simulink model "stable_ctime_v5"  (R2012b)
settings: Solver=VariableStepDiscrete  SolverMode=SingleTasking  StartTime=0.0  StopTime=10.0  RelTol=1e-3
undefined symbols (not defined in the file): pfb_coeff_gen_calc
libraries: xbsIndex_r4 x5705, casper_library_misc x63, casper_library_delays x27, casper_library_flow_control x20, xps_library x6
(part 2 of 68)

== system stable_ctime_v5/DAC_ADC ==
  i0 : Inport
  i1 : Inport  Port=2
  q0 : Inport  Port=3
  q1 : Inport  Port=4
  sync_iq : Inport  Port=5
  dac_reset : Inport  Port=6
  adc_mkid : xps_library/ADCs/adc_mkid  Tag=xps:adc_mkid  adc_brd=1  adc_clk_rate=512
  dac_mkid1 : Subsystem  Tag=xps:dac_mkid  AncestorBlock=xps_library/DACs/dac_mkid  mask(MKID DAC Interface Block){dac_brd=0, dac_clk_rate=512, sample_period=1}
      mask prompts: dac_brd "DAC board"; dac_clk_rate "DAC external clock rate (MHz)"; sample_period "Sample period"
      mask help: Interface block for the MKID 16-bits DAC board (2xDAC5681)
      mask init:
      | dac_mkid_mask;
      mask TypeOptions dac_brd: 0 | 1
  i0_adc : Outport
  i1_adc : Outport  Port=2
  q0_adc : Outport  Port=3
  q1_adc : Outport  Port=4
  sync : Outport  Port=5
  wires:
  i0/1 -> dac_mkid1/1(data_i0)
  i1/1 -> dac_mkid1/2(data_i1)
  q1/1 -> dac_mkid1/4(data_q1)
  adc_mkid/5 -> sync/1
  adc_mkid/2 -> i1_adc/1
  adc_mkid/4 -> q1_adc/1
  q0/1 -> dac_mkid1/3(data_q0)
  adc_mkid/3 -> q0_adc/1
  adc_mkid/1 -> i0_adc/1
  dac_reset/1 -> dac_mkid1/7(reset)
  sync_iq/1 -> dac_mkid1/6(sync_q), dac_mkid1/5(sync_i)

== system stable_ctime_v5/DDC ==
  note: latency = 8
  "sync_in " : Inport
  i0q0 : Inport  Port=2
  i1q1 : Inport  Port=3
  dds_delay : Inport  Port=4
  dds_i0 : Inport  Port=5
  "dds_q0 " : Inport  Port=6
  dds_i1 : Inport  Port=7
  dds_q1 : Inport  Port=8
  Delay{1,34..37} (5 alike) : xbsIndex_r4/Delay  rst=off  infoeditControl=Selection of Reset will increase slice count due to use of real FFs and instead of SRLs  en=off  latency=2  dbl_ovrd=off  reg_retiming=off  block_type=delay
  Delay2 : xbsIndex_r4/Delay  rst=off  infoeditControl=Selection of Reset will increase slice count due to use of real FFs and instead of SRLs  en=off  latency=8  dbl_ovrd=off  reg_retiming=off  block_type=delay
  c_to_ri3 : casper_library_misc/c_to_ri  n_bits=18  bin_pt=17
  c_to_ri6 : casper_library_misc/c_to_ri  n_bits=18  bin_pt=17
  delay_bram_prog : casper_library_delays/delay_bram_prog  MaxDelay=9  bram_latency=2
      link override AddSub: mode=Subtraction  use_carryin=off  use_carryout=off  en=off  latency=2  precision=User Defined  arith_type=Unsigned  n_bits=MaxDelay  bin_pt=0  quantization=Truncate  overflow=Wrap  dbl_ovrd=off  use_behavioral_HDL=off  hw_selection=DSP48  pipelined=on  use_rpm=on
      link override Counter: cnt_type=Free Running  cnt_to=inf  operation=Up  start_count=0  cnt_by_val=1  arith_type=Unsigned  n_bits=MaxDelay  bin_pt=0  load_pin=off  rst=on  en=off  explicit_period=on  period=1  dbl_ovrd=off  use_behavioral_HDL=off  implementation=DSP48  use_rpm=off
      link override Relational: mode=a>=b  en=off  latency=0  dbl_ovrd=off
      link override Single Port RAM: depth=2^MaxDelay  initVector=0  distributed_mem=Block RAM  write_mode=Read Before Write  rst=off  init_reg=0  en=off  latency=bram_latency  dbl_ovrd=off  optimize=Speed
      link override AddSub: xl_area=[0, 0, 0, 0, 0, 0, 0]
      link override Counter: infoedit="Hardware notes: Free running counters are the least expensive in hardware.  A count limited counter is implemented by combining a counter with a comparator."  xl_area=[0, 0, 0, 0, 0, 0, 0]
      link override Relational: xl_area=[0, 0, 0, 0, 0, 0, 0]
      link override Single Port RAM: xl_area=[0, 0, 0, 0, 0, 0, 0]
  delay_bram_prog1 : casper_library_delays/delay_bram_prog  MaxDelay=9  bram_latency=2
      link override AddSub: mode=Subtraction  use_carryin=off  use_carryout=off  en=off  latency=2  precision=User Defined  arith_type=Unsigned  n_bits=MaxDelay  bin_pt=0  quantization=Truncate  overflow=Wrap  dbl_ovrd=off  use_behavioral_HDL=off  hw_selection=DSP48  pipelined=on  use_rpm=on
      link override Counter: cnt_type=Free Running  cnt_to=inf  operation=Up  start_count=0  cnt_by_val=1  arith_type=Unsigned  n_bits=MaxDelay  bin_pt=0  load_pin=off  rst=on  en=off  explicit_period=on  period=1  dbl_ovrd=off  use_behavioral_HDL=off  implementation=DSP48  use_rpm=off
      link override Relational: mode=a>=b  en=off  latency=0  dbl_ovrd=off
      link override Single Port RAM: depth=2^MaxDelay  initVector=0  distributed_mem=Block RAM  write_mode=Read Before Write  rst=off  init_reg=0  en=off  latency=bram_latency  dbl_ovrd=off  optimize=Speed
      link override AddSub: xl_area=[0, 0, 0, 0, 0, 0, 0]
      link override Counter: infoedit="Hardware notes: Free running counters are the least expensive in hardware.  A count limited counter is implemented by combining a counter with a comparator."  xl_area=[0, 0, 0, 0, 0, 0, 0]
      link override Relational: xl_area=[0, 0, 0, 0, 0, 0, 0]
      link override Single Port RAM: xl_area=[0, 0, 0, 0, 0, 0, 0]
  delay_bram_prog2 : casper_library_delays/delay_bram_prog  MaxDelay=9  bram_latency=2
      link override AddSub: mode=Subtraction  use_carryin=off  use_carryout=off  en=off  latency=2  precision=User Defined  arith_type=Unsigned  n_bits=MaxDelay  bin_pt=0  quantization=Truncate  overflow=Wrap  dbl_ovrd=off  use_behavioral_HDL=off  hw_selection=DSP48  pipelined=on  use_rpm=on
      link override Counter: cnt_type=Free Running  cnt_to=inf  operation=Up  start_count=0  cnt_by_val=1  arith_type=Unsigned  n_bits=MaxDelay  bin_pt=0  load_pin=off  rst=on  en=off  explicit_period=on  period=1  dbl_ovrd=off  use_behavioral_HDL=off  implementation=DSP48  use_rpm=off
      link override Relational: mode=a>=b  en=off  latency=0  dbl_ovrd=off
      link override Single Port RAM: depth=2^MaxDelay  initVector=0  distributed_mem=Block RAM  write_mode=Read Before Write  rst=off  init_reg=0  en=off  latency=bram_latency  dbl_ovrd=off  optimize=Speed
      link override AddSub: xl_area=[0, 0, 0, 0, 0, 0, 0]
      link override Counter: infoedit="Hardware notes: Free running counters are the least expensive in hardware.  A count limited counter is implemented by combining a counter with a comparator."  xl_area=[0, 0, 0, 0, 0, 0, 0]
      link override Relational: xl_area=[0, 0, 0, 0, 0, 0, 0]
      link override Single Port RAM: xl_area=[0, 0, 0, 0, 0, 0, 0]
  delay_bram_prog3 : casper_library_delays/delay_bram_prog  MaxDelay=9  bram_latency=2
      link override AddSub: mode=Subtraction  use_carryin=off  use_carryout=off  en=off  latency=2  precision=User Defined  arith_type=Unsigned  n_bits=MaxDelay  bin_pt=0  quantization=Truncate  overflow=Wrap  dbl_ovrd=off  use_behavioral_HDL=off  hw_selection=DSP48  pipelined=on  use_rpm=on
      link override Counter: cnt_type=Free Running  cnt_to=inf  operation=Up  start_count=0  cnt_by_val=1  arith_type=Unsigned  n_bits=MaxDelay  bin_pt=0  load_pin=off  rst=on  en=off  explicit_period=on  period=1  dbl_ovrd=off  use_behavioral_HDL=off  implementation=DSP48  use_rpm=off
      link override Relational: mode=a>=b  en=off  latency=0  dbl_ovrd=off
      link override Single Port RAM: depth=2^MaxDelay  initVector=0  distributed_mem=Block RAM  write_mode=Read Before Write  rst=off  init_reg=0  en=off  latency=bram_latency  dbl_ovrd=off  optimize=Speed
      link override AddSub: xl_area=[0, 0, 0, 0, 0, 0, 0]
      link override Counter: infoedit="Hardware notes: Free running counters are the least expensive in hardware.  A count limited counter is implemented by combining a counter with a comparator."  xl_area=[0, 0, 0, 0, 0, 0, 0]
      link override Relational: xl_area=[0, 0, 0, 0, 0, 0, 0]
      link override Single Port RAM: xl_area=[0, 0, 0, 0, 0, 0, 0]
  mixer_even : Subsystem
  mixer_odd : Subsystem
  "sync_out " : Outport
  i0q0_out : Outport  Port=2
  i1q1_out : Outport  Port=3
  wires:
  i1q1/1 -> c_to_ri6/1
  i0q0/1 -> c_to_ri3/1
  dds_delay/1 -> delay_bram_prog1/2, delay_bram_prog3/2, delay_bram_prog2/2, delay_bram_prog/2
  c_to_ri3/1 -> Delay36/1
  c_to_ri3/2 -> Delay37/1
  c_to_ri6/1 -> Delay34/1
  c_to_ri6/2 -> Delay35/1
  dds_i0/1 -> delay_bram_prog/1
  delay_bram_prog/1 -> mixer_even/3(dds_I)
  "dds_q0 "/1 -> delay_bram_prog1/1
  dds_q1/1 -> delay_bram_prog3/1
  delay_bram_prog3/1 -> mixer_odd/4(dds_Q)
  delay_bram_prog1/1 -> mixer_even/4(dds_Q)
  Delay35/1 -> mixer_odd/2(data_Q)
  Delay34/1 -> mixer_odd/1(data_I)
  Delay36/1 -> mixer_even/1(data_I)
  Delay37/1 -> mixer_even/2(data_Q)
  delay_bram_prog2/1 -> mixer_odd/3(dds_I)
  mixer_even/1(mixed_out) -> i0q0_out/1
  mixer_odd/1(mixed_out) -> i1q1_out/1
  dds_i1/1 -> delay_bram_prog2/1
  "sync_in "/1 -> Delay1/1
  Delay1/1 -> Delay2/1
  Delay2/1 -> "sync_out "/1

== system stable_ctime_v5/DDC_snap ==
  note: 18.17 to 16.15
  sync_in : Inport
  i0q0_fft : Inport  Port=2
  i1q1_fft : Inport  Port=3
  i0q0_ddc : Inport  Port=4
  i1q1_ddc : Inport  Port=5
  dds_shift : Inport  Port=6
  dds_i0 : Inport  Port=7
  dds_q0 : Inport  Port=8
  dds_i1 : Inport  Port=9
  dds_q1 : Inport  Port=10
  Counter2 : xbsIndex_r4/Counter  cnt_type=Free Running  cnt_to=Inf  operation=Up  start_count=0  cnt_by_val=1  arith_type=Unsigned  n_bits=9  bin_pt=0  load_pin=off  rst=on  en=off  explicit_period=on  period=1  dbl_ovrd=off  use_behavioral_HDL=off  implementation=DSP48  block_type=counter
  Delay17 : xbsIndex_r4/Delay  rst=off  infoeditControl=Selection of Reset will increase slice count due to use of real FFs and instead of SRLs  en=off  latency=2  dbl_ovrd=off  reg_retiming=off  block_type=delay
  Delay25 : xbsIndex_r4/Delay  rst=off  infoeditControl=Selection of Reset will increase slice count due to use of real FFs and instead of SRLs  en=off  latency=2  dbl_ovrd=off  reg_retiming=off  block_type=delay
  Delay39 : xbsIndex_r4/Delay  rst=off  infoeditControl=Selection of Reset will increase slice count due to use of real FFs and instead of SRLs  en=off  latency=2  dbl_ovrd=off  reg_retiming=off  block_type=delay
  Delay42 : xbsIndex_r4/Delay  rst=off  infoeditControl=Selection of Reset will increase slice count due to use of real FFs and instead of SRLs  en=off  latency=8  dbl_ovrd=off  reg_retiming=off  block_type=delay
  Relational1 : xbsIndex_r4/Relational  mode=a=b  en=off  latency=0  dbl_ovrd=off  block_type=relational
  bus_create6 : Subsystem  AncestorBlock=casper_library_flow_control/bus_create  mask(bus_create){inputNum=4}
      mask prompts: inputNum "Number of inputs:"
      mask init:
      | bus_create_init(gcb,...
      |     'inputNum', inputNum);
  bus_create7 : Subsystem  AncestorBlock=casper_library_flow_control/bus_create  mask(bus_create){inputNum=2}
      mask prompts: inputNum "Number of inputs:"
      mask init:
      | bus_create_init(gcb,...
      |     'inputNum', inputNum);
  bus_create8 : Subsystem  AncestorBlock=casper_library_flow_control/bus_create  mask(bus_create){inputNum=2}
      mask prompts: inputNum "Number of inputs:"
      mask init:
      | bus_create_init(gcb,...
      |     'inputNum', inputNum);
  bus_create9 : Subsystem  AncestorBlock=casper_library_flow_control/bus_create  mask(bus_create){inputNum=2}
      mask prompts: inputNum "Number of inputs:"
      mask init:
      | bus_create_init(gcb,...
      |     'inputNum', inputNum);
  chan_select : Subsystem  Tag=xps:sw_reg  AncestorBlock=xps_library/software_register  mask(swreg){mode=one value, io_dir=From Processor, io_delay=0, sample_period=1, names=reg, bitwidths=32, arith_types=0, bin_pts=0, sim_port=off, show_format=off}
      mask prompts: io_dir "I/O direction"; io_delay "I/O delay"; sample_period "Sample period"; names "Name:"; bitwidths "Bitwidth:"; arith_types "Type (ufix=0, fix=1, bool=2):"; bin_pts "Binary pt:"; sim_port "Provide sim input/output?"; show_format "Print format string?"
      mask init:
      | swreg_init(gcb)
      settings: AttributesFormatString=1input
      mask TypeOptions mode: one value | fields of equal size | fields of arbitrary size
      mask Callback mode: swreg_cb(gcb);
      mask TypeOptions io_dir: To Processor | From Processor
      mask Callback io_dir:
      | mask_enables = get_param(gcb, 'MaskEnables');
      | mask_names = get_param(gcb, 'MaskNames');
      | if strcmp(get_param(gcb, 'io_dir'), 'To Processor'),
      |     mask_enables{ismember(mask_names, 'sample_period')} = 'off';
      | else
      |     mask_enables{ismember(mask_names, 'sample_period')} = 'on';
      | end
      | set_param(gcb, 'MaskEnables', mask_enables);
      mask Callback bitwidths:
      | swreg_maskcheck(gcb);
      | % blk = gcb;
      | % mode = get_param(blk, 'mode');
      | % current_widths = eval(get_param(blk, 'bitwidths'));
      | % if (strcmp(mode, 'one value') || strcmp(mode, 'fields of equal size')) && (length(current_widths) > 1),
      | %     error('Only one width may be specified for this mode.');
      | % elseif strcmp(mode, 'fields of arbitrary size')
      | %     current_names = textscan(strtrim(strrep(strrep(get_param(blk, 'names'), ']', ''), '[', '')), '%s');
      | %     current_names = current_names{1};
      | %     numios = length(current_names);
      | %     if length(current_widths) ~= numios,
      | %         error('%d field names specified, but %d widths?', numios, length(current_widths));
      | %     end
      | % end
      | % total_width = 0;
      | % for ctr = 1 : length(current_widths),
      | %     total_width = total_width + current_widths(ctr);
      | % end
      | % if total_width > 32,
      | %     error('Total width must be 32 or less, set to %d.', total_width);
      | % end
      mask Callback arith_types:
      | [numios, ~, ~, ~, current_types] = swreg_maskcheck(gcb);
      | % blk = gcb;
      | % mode = get_param(blk, 'mode');
      | % current_types = eval(get_param(blk, 'arith_types'));
      | % numios = length(current_types);
      | % if (strcmp(mode, 'one value') || strcmp(mode, 'fields of equal size')) && (length(current_types) > 1),
      | %     error('Only one type may be specified for this mode.');
      | % elseif strcmp(mode, 'fields of arbitrary size')
      | %     current_names = textscan(strtrim(strrep(strrep(get_param(blk, 'names'), ']', ''), '[', '')), '%s');
      | %     current_names = current_names{1};
      | %     numios = length(current_names);
      | %     if length(current_types) ~= numios,
      | %         error('%d field names specified, but %d types?', numios, length(current_types));
      | %     end
      | % end
      | problem = 0;
      | for ctr = 1 : numios,
      |     t = current_types(ctr);
      |     if (t < 0) || (t > 2),
      |         problem = t;
      |         ctr = numios + 1;
      |     end
      | end
      | if problem ~= 0,
      |     error('Type cannot be %i, must be 0, 1 or 2.', problem);
      | end
      mask Callback bin_pts:
      | swreg_maskcheck(gcb);
      | % blk = gcb;
      | % mode = get_param(blk, 'mode');
      | % current_bins = eval(get_param(blk, 'bin_pts'));
      | % if (strcmp(mode, 'one value') || strcmp(mode, 'fields of equal size')) && (length(current_bins) > 1),
      | %     error('Only one binary pt may be specified for this mode.');
      | % elseif strcmp(mode, 'fields of arbitrary size')
      | %     current_names = textscan(strtrim(strrep(strrep(get_param(blk, 'names'), ']', ''), '[', '')), '%s');
      | %     current_names = current_names{1};
      | %     numios = length(current_names);
      | %     if length(current_bins) ~= numios,
      | %         error('%d field names specified, but %d binary pts?', numios, length(current_bins));
      | %     end
      | % end
  delay_bram_prog : casper_library_delays/delay_bram_prog  MaxDelay=9  bram_latency=2
      link override AddSub: mode=Subtraction  use_carryin=off  use_carryout=off  en=off  latency=2  precision=User Defined  arith_type=Unsigned  n_bits=MaxDelay  bin_pt=0  quantization=Truncate  overflow=Wrap  dbl_ovrd=off  use_behavioral_HDL=off  hw_selection=DSP48  pipelined=on  use_rpm=on
      link override Counter: cnt_type=Free Running  cnt_to=inf  operation=Up  start_count=0  cnt_by_val=1  arith_type=Unsigned  n_bits=MaxDelay  bin_pt=0  load_pin=off  rst=on  en=off  explicit_period=on  period=1  dbl_ovrd=off  use_behavioral_HDL=off  implementation=DSP48  use_rpm=off
      link override Relational: mode=a>=b  en=off  latency=0  dbl_ovrd=off
      link override Single Port RAM: depth=2^MaxDelay  initVector=0  distributed_mem=Block RAM  write_mode=Read Before Write  rst=off  init_reg=0  en=off  latency=bram_latency  dbl_ovrd=off  optimize=Speed
      link override AddSub: xl_area=[0, 0, 0, 0, 0, 0, 0]
      link override Counter: infoedit="Hardware notes: Free running counters are the least expensive in hardware.  A count limited counter is implemented by combining a counter with a comparator."  xl_area=[0, 0, 0, 0, 0, 0, 0]
      link override Relational: xl_area=[0, 0, 0, 0, 0, 0, 0]
      link override Single Port RAM: xl_area=[0, 0, 0, 0, 0, 0, 0]
  delay_bram_prog1 : casper_library_delays/delay_bram_prog  MaxDelay=9  bram_latency=2
      link override AddSub: mode=Subtraction  use_carryin=off  use_carryout=off  en=off  latency=2  precision=User Defined  arith_type=Unsigned  n_bits=MaxDelay  bin_pt=0  quantization=Truncate  overflow=Wrap  dbl_ovrd=off  use_behavioral_HDL=off  hw_selection=DSP48  pipelined=on  use_rpm=on
      link override Counter: cnt_type=Free Running  cnt_to=inf  operation=Up  start_count=0  cnt_by_val=1  arith_type=Unsigned  n_bits=MaxDelay  bin_pt=0  load_pin=off  rst=on  en=off  explicit_period=on  period=1  dbl_ovrd=off  use_behavioral_HDL=off  implementation=DSP48  use_rpm=off
      link override Relational: mode=a>=b  en=off  latency=0  dbl_ovrd=off
      link override Single Port RAM: depth=2^MaxDelay  initVector=0  distributed_mem=Block RAM  write_mode=Read Before Write  rst=off  init_reg=0  en=off  latency=bram_latency  dbl_ovrd=off  optimize=Speed
      link override AddSub: xl_area=[0, 0, 0, 0, 0, 0, 0]
      link override Counter: infoedit="Hardware notes: Free running counters are the least expensive in hardware.  A count limited counter is implemented by combining a counter with a comparator."  xl_area=[0, 0, 0, 0, 0, 0, 0]
      link override Relational: xl_area=[0, 0, 0, 0, 0, 0, 0]
      link override Single Port RAM: xl_area=[0, 0, 0, 0, 0, 0, 0]
  downselect18to16 : Subsystem
  downselect18to2 : Subsystem
  downselect19to1 : Subsystem
  downselect19to2 : Subsystem
  mixerout : Subsystem  Tag=casper:snapshot  AncestorBlock=casper_library_scopes/snapshot  mask(snapshot){storage=bram, dram_dimm=1, dram_clock=200, nsamples=14, data_width=64, offset=off, circap=off, value=off, use_dsp48=on}
      mask prompts: storage "Storage medium"; dram_dimm "DRAM dimm"; dram_clock "DRAM clock rate"; nsamples "Number of Samples (2^?)"; data_width "Data width"; offset "Start delay support"; circap "Circular capture support"; value "Extra value capture support"; use_dsp48 "Use DSP48s to implement counters"
      mask help:
      | Standard snap block, but with the following optional extras;
      |  1) Optionally delay the fabric trigger by a user-specified number of valids.
      |  2) Capture continuously after a trigger until a stop pulse is received. Data is captured into BRAM continuously, with old data being overwritten until a stop command is received. Then stop capturing when memory is filled. This enables you to get some data before and some data after the stop pulse. Use the 'tr_en_cnt' register to determine where you are in your vector. 'Addr' register's MSb now indicates 'busy capturing'.
      |  3) Optionally capture a value on an input port to a register at the same time as the first data sample.
      |  4) Implement counters using DSP48Es to save resources.
      mask init:
      | snapshot_init(gcb, ...
      |     'storage', storage, ...
      |     'dram_dimm', dram_dimm, ...
      |     'dram_clock', dram_clock, ...
      |     'nsamples', nsamples, ...
      |     'data_width', data_width, ...
      |     'offset', offset, ...
      |     'circap', circap, ...
      |     'value', value, ...
      |     'use_dsp48', use_dsp48);
      mask TypeOptions storage: bram | dram
      mask Callback storage: snapshot_callback();
      mask TypeOptions dram_dimm: 1 | 2 | 3 | 4
      mask TypeOptions dram_clock: 200 | 250 | 266 | 300 | 333
      mask TypeOptions data_width: 8 | 16 | 32 | 64 | 128
  rawfftbin : Subsystem  Tag=casper:snapshot  AncestorBlock=casper_library_scopes/snapshot  mask(snapshot){storage=bram, dram_dimm=1, dram_clock=200, nsamples=14, data_width=128, offset=off, circap=off, value=off, use_dsp48=on}
      mask prompts: storage "Storage medium"; dram_dimm "DRAM dimm"; dram_clock "DRAM clock rate"; nsamples "Number of Samples (2^?)"; data_width "Data width"; offset "Start delay support"; circap "Circular capture support"; value "Extra value capture support"; use_dsp48 "Use DSP48s to implement counters"
      mask help:
      | Standard snap block, but with the following optional extras;
      |  1) Optionally delay the fabric trigger by a user-specified number of valids.
      |  2) Capture continuously after a trigger until a stop pulse is received. Data is captured into BRAM continuously, with old data being overwritten until a stop command is received. Then stop capturing when memory is filled. This enables you to get some data before and some data after the stop pulse. Use the 'tr_en_cnt' register to determine where you are in your vector. 'Addr' register's MSb now indicates 'busy capturing'.
      |  3) Optionally capture a value on an input port to a register at the same time as the first data sample.
      |  4) Implement counters using DSP48Es to save resources.
      mask init: same as stable_ctime_v5/DDC_snap/mixerout
      mask TypeOptions storage: bram | dram
      mask Callback storage: snapshot_callback();
      mask TypeOptions dram_dimm: 1 | 2 | 3 | 4
      mask TypeOptions dram_clock: 200 | 250 | 266 | 300 | 333
      mask TypeOptions data_width: 8 | 16 | 32 | 64 | 128
  wires:
  i1q1_fft/1 -> downselect18to2/1(ComplexIn)
  i1q1_ddc/1 -> downselect19to2/1(ComplexIn)
  i0q0_ddc/1 -> downselect19to1/1(ComplexIn)
  dds_shift/1 -> delay_bram_prog1/2, delay_bram_prog/2
  Counter2/1 -> Relational1/2
  downselect18to16/1(Out1) -> Delay17/1
  downselect18to2/1(Out1) -> Delay25/1
  dds_i0/1 -> bus_create7/1(in1)
  dds_q0/1 -> bus_create7/2(in2)
  dds_i1/1 -> bus_create8/1(in1)
  dds_q1/1 -> bus_create8/2(in2)
  downselect19to1/1(Out1) -> bus_create9/1(in1)
  downselect19to2/1(Out1) -> bus_create9/2(in2)
  bus_create9/1(bus_out) -> mixerout/1(din)
  delay_bram_prog/1 -> bus_create6/2(in2)
  bus_create7/1(bus_out) -> delay_bram_prog/1
  bus_create8/1(bus_out) -> delay_bram_prog1/1
  delay_bram_prog1/1 -> bus_create6/4(in4)
  Delay17/1 -> bus_create6/1(in1)
  Delay25/1 -> bus_create6/3(in3)
  Delay42/1 -> mixerout/3(trig), mixerout/2(we)
  Relational1/1 -> Delay39/1
  Delay39/1 -> rawfftbin/3(trig), rawfftbin/2(we), Delay42/1
  i0q0_fft/1 -> downselect18to16/1(ComplexIn)
  chan_select/1(in_reg) -> Relational1/1
  sync_in/1 -> Counter2/1
  bus_create6/1(bus_out) -> rawfftbin/1(din)
